simulink subsystem "s0320_alpha_theta_PP"  (R2019b)
settings: Solver=VariableStepAuto  StartTime=0.0  StopTime=10.0  RelTol=1e-3
undefined symbols (not defined in the file): den_der_filter, dt_control, num_der_filter
settings Model: Creator=francescoceresetti  LastModifiedBy=paolo

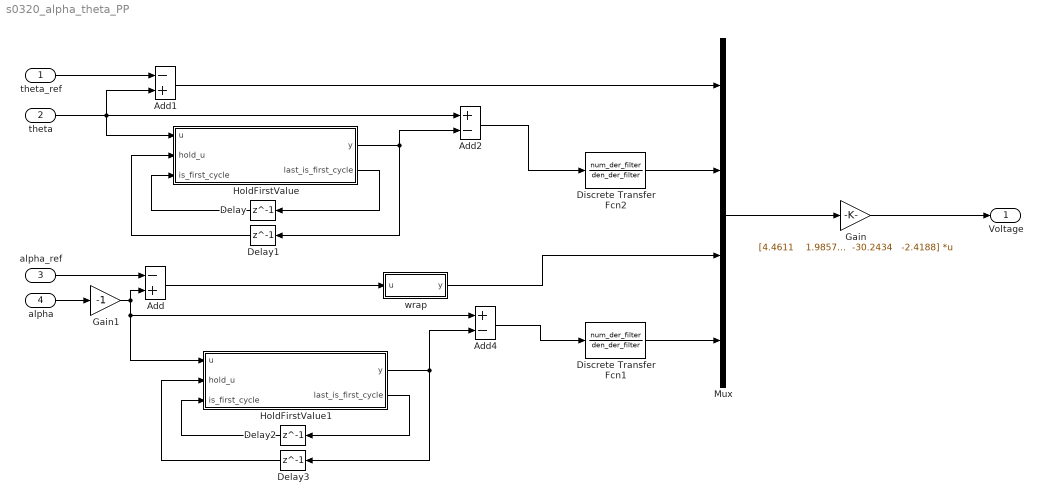
== system s0320_alpha_theta_PP ==
  theta_ref : Inport
  theta : Inport  Port=2
  alpha_ref : Inport  Port=3
  alpha : Inport  Port=4
  Add : Sum  Inputs=-+
  Add1 : Sum  Inputs=-+
  Add2 : Sum  Inputs=+-
  Add4 : Sum  Inputs=+-
  Delay{,1..3} (4 alike) : Delay  DelayLength=1  InitialCondition=1
  Discrete Transfer Fcn1 : DiscreteTransferFcn  Numerator=num_der_filter  Denominator=den_der_filter  SampleTime=dt_control
  Discrete Transfer Fcn2 : DiscreteTransferFcn  Numerator=num_der_filter  Denominator=den_der_filter  SampleTime=dt_control
  Gain : Gain  Gain="[4.4611    1.9857  -30.2434   -2.4188]"  Multiplication=Matrix(K*u)
  Gain1 : Gain  Gain=-1
  HoldFirstValue : MATLAB Function  TreatAsAtomicUnit=on
  HoldFirstValue1 : MATLAB Function  TreatAsAtomicUnit=on
  Mux : Mux
  wrap : MATLAB Function  TreatAsAtomicUnit=on
  Voltage : Outport
  wires:
  theta_ref/1 -> Add1/1
  alpha/1 -> Gain1/1
  Mux/1 -> Gain/1
  Gain/1 -> Voltage/1
  Add1/1 -> Mux/1
  theta/1 -> Add1/2, Add2/1, HoldFirstValue/1(u)
  alpha_ref/1 -> Add/1
  Gain1/1 -> Add/2, Add4/1, HoldFirstValue1/1(u)
  Discrete Transfer Fcn1/1 -> Mux/4
  HoldFirstValue/2(last_is_first_cycle) -> Delay/1
  Delay/1 -> HoldFirstValue/3(is_first_cycle)
  HoldFirstValue/1(y) -> Delay1/1, Add2/2
  Delay1/1 -> HoldFirstValue/2(hold_u)
  Add2/1 -> Discrete Transfer Fcn2/1
  Discrete Transfer Fcn2/1 -> Mux/2
  HoldFirstValue1/2(last_is_first_cycle) -> Delay2/1
  Delay2/1 -> HoldFirstValue1/3(is_first_cycle)
  HoldFirstValue1/1(y) -> Delay3/1, Add4/2
  Delay3/1 -> HoldFirstValue1/2(hold_u)
  Add/1 -> wrap/1(u)
  Add4/1 -> Discrete Transfer Fcn1/1
  wrap/1(y) -> Mux/3

== matlab function s0320_alpha_theta_PP/HoldFirstValue ==
  data: u input; y output; hold_u input; is_first_cycle input; last_is_first_cycle output
function [y,last_is_first_cycle]  = holdFirstValue(u, hold_u, is_first_cycle)

if is_first_cycle
    y = u;
else
    y = hold_u;
end
last_is_first_cycle = 0;

end

== matlab function s0320_alpha_theta_PP/HoldFirstValue1 ==
  data: u input; y output; hold_u input; is_first_cycle input; last_is_first_cycle output
function [y,last_is_first_cycle]  = holdFirstValue(u, hold_u, is_first_cycle)

if is_first_cycle
    y = u;
else
    y = hold_u;
end
last_is_first_cycle = 0;

end

== matlab function s0320_alpha_theta_PP/wrap ==
  data: u input; y output
function y = wrap(u)
stop_condition = false;
y = u;
while ~stop_condition
    if y > pi
        y = y - 2*pi;
    elseif y < -pi
        y = y + 2*pi;
    else
        stop_condition = true;
    end
end
